simulink model "spectrum_analyzer_1"  (R2021b)
settings: Solver=VariableStepAuto  StartTime=0.0  StopTime=5  RelTol=1e-3
libraries: dspsnks4 x1
settings Model: Creator=paulom  LastModifiedBy=paulom

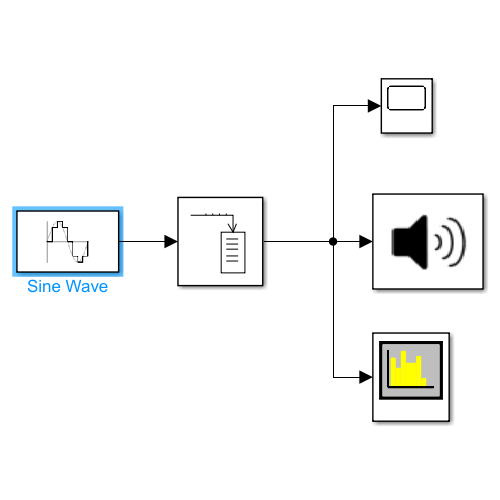
[thumbnail: Simulink's stored preview of the top-level diagram]
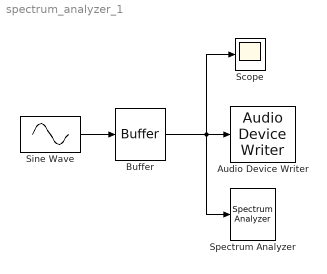
== system spectrum_analyzer_1 ==
  Audio Device Writer : dspsnks4/Audio Device Writer  Driver=DirectSound  Device=Default  InheritSampleRate=off  SampleRate=44100  BitDepth=16-bit integer  BufferSize=4096  NumBuffers=10  DefaultOutputChannelMapping=on  OutputChannelMapping=1:2  OutputNumUnderrunSamples=off  DriverIdx=1  DeviceWarnFlag=''
  Buffer : Buffer  N=1024  OutputFrames=off
  Scope : Scope
  Sine Wave : Sin  Frequency=2*pi*100  SampleTime=1/44100
  Spectrum Analyzer : SpectrumAnalyzer
  wires:
  Sine Wave/1 -> Buffer/1
  Buffer/1 -> Audio Device Writer/1, Scope/1, Spectrum Analyzer/1
